simulink model "EPD629_WilliamsJ_AS08_Simulink"  (R2021b)
settings: Solver=VariableStepAuto  StartTime=0.0  StopTime=70  MaxStep=.02  RelTol=1e-3
values from neighbouring files (symbols this model uses):
  AirGasConstant_kJpkgK = 0.287    [EPD629_WilliamsJ_AS08.m]
  AirToFuelEquivalenceRatio_frac = 1    [EPD629_WilliamsJ_AS08.m]
  AmbientPressure_kPa = 98    [EPD629_WilliamsJ_AS08.m]
  BaseSparkAdvanceData_deg = min(MBTSparkAdvanceData_deg,BorderlineSparkAdvData_deg)    [EPD629_WilliamsJ_AS08.m]
  CrankAngleIVCToTDC_deg = 170    [EPD629_WilliamsJ_AS08.m]
  CylinderAirMassBreakpoints_mg = 0:25:400    [EPD629_WilliamsJ_AS08.m]
  DelayFuelInjectionToIVC_rev = 0.75    [EPD629_WilliamsJ_AS08.m]
  DelayFuelInjectionToIVCEst_rev = 0.75    [EPD629_WilliamsJ_AS08.m]
  DelayIVCToOxygenSensor_rev = 7    [EPD629_WilliamsJ_AS08.m]
  DischargeCoefficient_frac = 0.7    [EPD629_WilliamsJ_AS08.m]
  EngineDisplacement_L = 2.77    [EPD629_WilliamsJ_AS08.m]
  EngineInertia_kgm2 = 0.2    [EPD629_WilliamsJ_AS08.m]
  EngineMotoringFrictionData_Nm = Beta_0 + Beta_2*Omega_e.^2    [EPD629_WilliamsJ_AS08.m]
  EngineSpeedBreakpoints_rpm = 400:200:5000    [EPD629_WilliamsJ_AS08.m]
  FuelControlIntegralGain = 2e-5    (= 2e-05)    [EPD629_WilliamsJ_AS08.m]
  FuelControlProportionalGain = 5e-6    (= 5e-06)    [EPD629_WilliamsJ_AS08.m]
  FuelInjEvapTimeConstant_s = 0.8    [EPD629_WilliamsJ_AS08.m]
  FuelInjEvapTimeConstantEst_s = 0.8    [EPD629_WilliamsJ_AS08.m]
  FuelInjImpactFactor_frac = 0.3    [EPD629_WilliamsJ_AS08.m]
  FuelInjImpactFactorEst_frac = 0.3    [EPD629_WilliamsJ_AS08.m]
  FuelLowerHeatingValue_kJpkg = 44000    [EPD629_WilliamsJ_AS08.m]
  InletAirTemperature_K = 298    [EPD629_WilliamsJ_AS08.m]
  IntakeManifoldVolume_L = 5.8    [EPD629_WilliamsJ_AS08.m]
  ManifoldAirTemperature_K = 340    [EPD629_WilliamsJ_AS08.m]
  ManifoldPressureBreakpoints_kPa = 5:5:100    [EPD629_WilliamsJ_AS08.m]
  NumberOfCylinders = 6    [EPD629_WilliamsJ_AS08.m]
  OxygenSensorLambdaBP_frac = [0 0.9 0.92 0.94 0.96 0.985 0.999 1.001 1.015 1.04 1.06 1.08 1.1 2]    [EPD629_WilliamsJ_AS08.m]
  OxygenSensorSwitchSetpoint_mV = 450    [EPD629_WilliamsJ_AS08.m]
  OxygenSensorVoltageData_mV = [800 800 794 788 775 750 700 200 150 125 112 106 100 100]    [EPD629_WilliamsJ_AS08.m]
  SparkTorqFactorData_frac = 1 - (SparkTorqFactorRetFromMBTBP_deg.^2) /      (SparkTorqFactorRetFromMBTBP_deg(end)^2)    [EPD629_WilliamsJ_AS08.m]
  SparkTorqFactorRetFromMBTBP_deg = 0:5:45    [EPD629_WilliamsJ_AS08.m]
  StoichiometricAFR_frac = 14.7    [EPD629_WilliamsJ_AS08.m]
  ThermodynamicEfficiencyData_frac = Eta_0 + Eta_1*Omega_e + Eta_2*Omega_e.^2    [EPD629_WilliamsJ_AS08.m]
  ThrottleAreaBreakpoints_pct = ThrottleAreaData_pct    [EPD629_WilliamsJ_AS08.m]
  ThrottleAreaData_pct = 100 * ThrottleArea_mm2 / WideOpenThrottleArea_mm2    [EPD629_WilliamsJ_AS08.m]
  ThrottleFlowFunctionData_frac = PR.^(1/RatioOfSpecificHeats_frac) .*      sqrt( 2 * RatioOfSpecificHeats_frac / (RatioOfSpecificHeats_frac - 1) .*      (1 - PR.^((RatioOfSpecificHeats_frac - 1) / RatioOfSpecificHeats_frac)) )    [EPD629_WilliamsJ_AS08.m]
  ThrottleMassFlowCorrIntGain = 10    [EPD629_WilliamsJ_AS08.m]
  ThrottlePositionBreakpoints_pct = 0:100    [EPD629_WilliamsJ_AS08.m]
  ThrottlePositionData_pct = ThrottlePositionBreakpoints_pct    [EPD629_WilliamsJ_AS08.m]
  ThrottlePressureRatioBreakpoints_frac = 0:0.01:1    [EPD629_WilliamsJ_AS08.m]
  VECorrectionFactorIntGain = 0.02    [EPD629_WilliamsJ_AS08.m]
  WideOpenThrottleArea_mm2 = ThrottleArea_mm2(end)    [EPD629_WilliamsJ_AS08.m]
undefined symbols (not defined in the file or in its folder): MBTSparkAdvanceData_deg, SparkTorqFactorBreakpoints_frac, SparkTorqFactorRetFromMBTData_deg, VolumetricEfficiencyData_frac
(part 2 of 2)

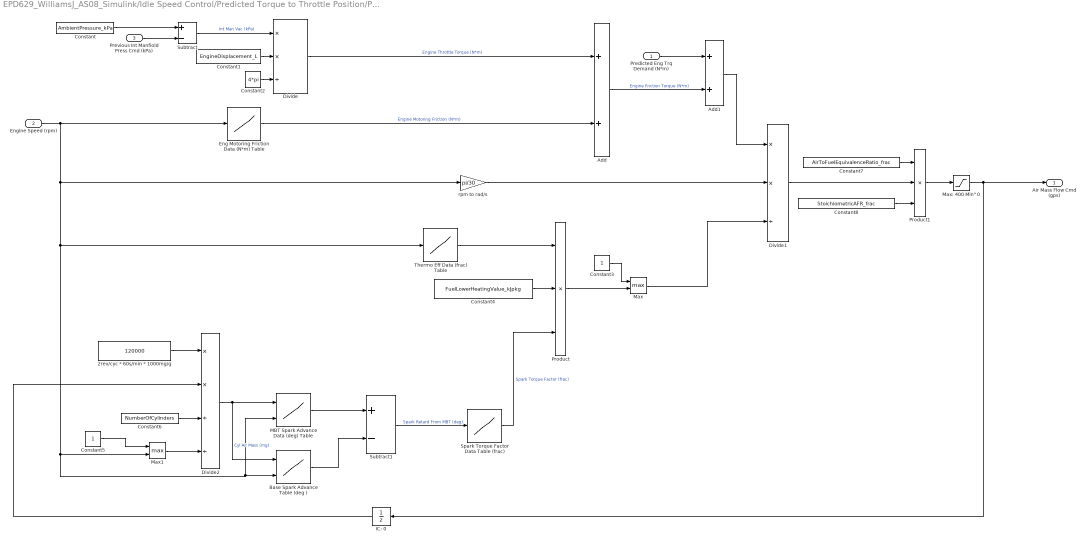
== system EPD629_WilliamsJ_AS08_Simulink/Idle Speed Control/Predicted Torque to Throttle Position/Predicted Torque to Air Mass Flow ==
  Predicted Eng Trq Demand (N*m) : Inport
  Engine Speed (rpm) : Inport  Port=2
  Previous Int Manfiold Press Cmd (kPa) : Inport  Port=3
  2rev/cyc * 60s/min * 1000mg/g : Constant  Value=120000
  Add : Sum
  Add1 : Sum
  Base Spark Advance Table (deg ) : Lookup_n-D  BreakpointsForDimension1=CylinderAirMassBreakpoints_mg  BreakpointsForDimension2=EngineSpeedBreakpoints_rpm  Table=BaseSparkAdvanceData_deg  ExtrapMethod=Clip  UseLastTableValue=on  InternalRulePriority=Speed  RndMeth=Simplest  InputSameDT=on
      settings: InputPortMap=u0,u1
  Constant : Constant  Value=AmbientPressure_kPa
  Constant1 : Constant  Value=EngineDisplacement_L
  Constant2 : Constant  Value=4*pi
  Constant3 : Constant
  Constant4 : Constant  Value=FuelLowerHeatingValue_kJpkg
  Constant5 : Constant
  Constant6 : Constant  Value=NumberOfCylinders
  Constant7 : Constant  Value=AirToFuelEquivalenceRatio_frac
  Constant8 : Constant  Value=StoichiometricAFR_frac
  Divide : Product  Inputs=**/
  Divide1 : Product  Inputs=**/
  Divide2 : Product  Inputs=**//
  Eng Motoring Friction Data (N*m) Table : Lookup_n-D  NumberOfTableDimensions=1  BreakpointsForDimension1=EngineSpeedBreakpoints_rpm  Table=EngineMotoringFrictionData_Nm  ExtrapMethod=Clip  UseLastTableValue=on  InternalRulePriority=Speed  RndMeth=Simplest  InputSameDT=on
  IC: 0 : UnitDelay  SampleTime=-1  HasFrameUpgradeWarning=on
  MBT Spark Advance Data (deg) Table : Lookup_n-D  BreakpointsForDimension1=CylinderAirMassBreakpoints_mg  BreakpointsForDimension2=EngineSpeedBreakpoints_rpm  Table=MBTSparkAdvanceData_deg  ExtrapMethod=Clip  UseLastTableValue=on  InternalRulePriority=Speed  RndMeth=Simplest  InputSameDT=on
      settings: InputPortMap=u0,u1
  Max : MinMax  Function=max  Inputs=2
  Max1 : MinMax  Function=max  Inputs=2
  "Max: 400 Min\" 0" : Saturate  UpperLimit=400  LowerLimit=0
  Product : Product  Inputs=3
  Product1 : Product  Inputs=3
  Spark Torque Factor Data Table (frac) : Lookup_n-D  NumberOfTableDimensions=1  BreakpointsForDimension1=SparkTorqFactorRetFromMBTBP_deg  Table=SparkTorqFactorData_frac  ExtrapMethod=Clip  UseLastTableValue=on  InternalRulePriority=Speed  RndMeth=Simplest  InputSameDT=on
  Subtract : Sum  Inputs=+-
  Subtract1 : Sum  Inputs=+-
  Thermo Eff Data (frac) Table : Lookup_n-D  NumberOfTableDimensions=1  BreakpointsForDimension1=EngineSpeedBreakpoints_rpm  Table=ThermodynamicEfficiencyData_frac  ExtrapMethod=Clip  UseLastTableValue=on  InternalRulePriority=Speed  RndMeth=Simplest  InputSameDT=on
  rpm to rad/s : Gain  Gain=pi/30
  Air Mass Flow Cmd (gps) : Outport
  wires:
  Previous Int Manfiold Press Cmd (kPa)/1 -> Subtract/2
  Constant/1 -> Subtract/1
  Subtract/1 -> Divide/1  "Int Man Vac (kPa)"
  Constant1/1 -> Divide/2
  Constant2/1 -> Divide/3
  Divide/1 -> Add/1  "Engine Throttle Torque (N*m)"
  Engine Speed (rpm)/1 -> rpm to rad/s/1, Thermo Eff Data (frac) Table/1, Max1/2, MBT Spark Advance Data (deg) Table/2, Base Spark Advance Table (deg )/2, Eng Motoring Friction Data (N*m) Table/1
  Eng Motoring Friction Data (N*m) Table/1 -> Add/2  "Engine Motoring Friction (N*m)"
  rpm to rad/s/1 -> Divide1/2
  Thermo Eff Data (frac) Table/1 -> Product/1
  Product/1 -> Max/2
  Constant3/1 -> Max/1
  Max/1 -> Divide1/3
  Constant4/1 -> Product/2
  Constant5/1 -> Max1/1
  Max1/1 -> Divide2/4
  Constant6/1 -> Divide2/3
  2rev/cyc * 60s/min * 1000mg/g/1 -> Divide2/1
  Divide1/1 -> Product1/2
  Constant7/1 -> Product1/1
  Constant8/1 -> Product1/3
  Product1/1 -> "Max: 400 Min\" 0"/1
  "Max: 400 Min\" 0"/1 -> IC: 0/1, Air Mass Flow Cmd (gps)/1
  IC: 0/1 -> Divide2/2
  Divide2/1 -> MBT Spark Advance Data (deg) Table/1, Base Spark Advance Table (deg )/1  "Cyl Air Mass (mg)"
  MBT Spark Advance Data (deg) Table/1 -> Subtract1/1
  Base Spark Advance Table (deg )/1 -> Subtract1/2
  Subtract1/1 -> Spark Torque Factor Data Table (frac)/1  "Spark Retard From MBT (deg)"
  Spark Torque Factor Data Table (frac)/1 -> Product/3  "Spark Torque Factor (frac)"
  Predicted Eng Trq Demand (N*m)/1 -> Add1/1
  Add/1 -> Add1/2  "Engine Friction Torque (N*m)"
  Add1/1 -> Divide1/1

== system EPD629_WilliamsJ_AS08_Simulink/SparkAndFuelControl/Spark Advance Control/Spark Advance Calculation ==
  Spark Retard from MBT (deg) : Inport
  Engine Speed (rpm) : Inport  Port=2
  SpeedDensityMassFlowEst_gps : Inport  Port=3
  Base Spark Advance Data (deg) Table : Lookup_n-D  BreakpointsForDimension1=CylinderAirMassBreakpoints_mg  BreakpointsForDimension2=EngineSpeedBreakpoints_rpm  Table=BaseSparkAdvanceData_deg  ExtrapMethod=Clip  UseLastTableValue=on  InternalRulePriority=Speed  RndMeth=Simplest  InputSameDT=on
      settings: InputPortMap=u0,u1
  Constant : Constant  Value=120000
  Constant1 : Constant  Value=NumberOfCylinders
  Constant2 : Constant
  Divide : Product  Inputs=**//
  MBT Spark Advance Data (deg) Table : Lookup_n-D  BreakpointsForDimension1=CylinderAirMassBreakpoints_mg  BreakpointsForDimension2=EngineSpeedBreakpoints_rpm  Table=MBTSparkAdvanceData_deg  ExtrapMethod=Clip  UseLastTableValue=on  InternalRulePriority=Speed  RndMeth=Simplest  InputSameDT=on
      settings: InputPortMap=u0,u1
  Max : MinMax  Function=max  Inputs=2
  Min : MinMax  Inputs=2
  Subtract : Sum  Inputs=+-
  Spark Advance (deg) : Outport
  wires:
  Engine Speed (rpm)/1 -> MBT Spark Advance Data (deg) Table/2, Base Spark Advance Data (deg) Table/2, Max/2
  Constant1/1 -> Divide/3
  Constant2/1 -> Max/1
  SpeedDensityMassFlowEst_gps/1 -> Divide/2
  Constant/1 -> Divide/1  "2rev/cyc * 60sec/min * 1000 mg/g"
  Max/1 -> Divide/4
  Base Spark Advance Data (deg) Table/1 -> Min/1  "Base Spark Advance (deg)"
  Divide/1 -> MBT Spark Advance Data (deg) Table/1, Base Spark Advance Data (deg) Table/1  "Cyl Air Mass (mg)"
  MBT Spark Advance Data (deg) Table/1 -> Subtract/1
  Spark Retard from MBT (deg)/1 -> Subtract/2
  Subtract/1 -> Min/2  "Spark Advance Max (deg)"
  Min/1 -> Spark Advance (deg)/1

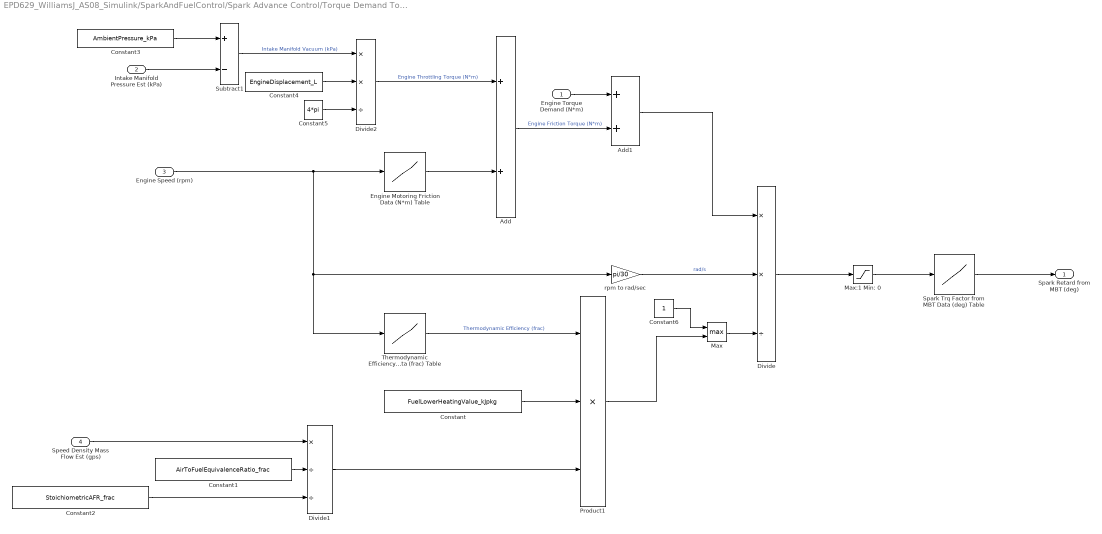
== system EPD629_WilliamsJ_AS08_Simulink/SparkAndFuelControl/Spark Advance Control/Torque Demand To Spark Retard from MBT ==
  Engine Torque Demand (N*m) : Inport
  Intake Manifold Pressure Est (kPa) : Inport  Port=2
  Engine Speed (rpm) : Inport  Port=3
  Speed Density Mass Flow Est (gps) : Inport  Port=4
  Add : Sum
  Add1 : Sum
  Constant : Constant  Value=FuelLowerHeatingValue_kJpkg
  Constant1 : Constant  Value=AirToFuelEquivalenceRatio_frac
  Constant2 : Constant  Value=StoichiometricAFR_frac
  Constant3 : Constant  Value=AmbientPressure_kPa
  Constant4 : Constant  Value=EngineDisplacement_L
  Constant5 : Constant  Value=4*pi
  Constant6 : Constant
  Divide : Product  Inputs=**/
  Divide1 : Product  Inputs=*//
  Divide2 : Product  Inputs=**/
  Engine Motoring Friction Data (N*m) Table : Lookup_n-D  NumberOfTableDimensions=1  BreakpointsForDimension1=EngineSpeedBreakpoints_rpm  Table=EngineMotoringFrictionData_Nm  ExtrapMethod=Clip  UseLastTableValue=on  InternalRulePriority=Speed  RndMeth=Simplest  InputSameDT=on
  Max : MinMax  Function=max  Inputs=2
  Max:1 Min: 0 : Saturate  UpperLimit=1  LowerLimit=0
  Product1 : Product  Inputs=3
  Spark Trq Factor from MBT Data (deg) Table : Lookup_n-D  NumberOfTableDimensions=1  BreakpointsForDimension1=SparkTorqFactorBreakpoints_frac  Table=SparkTorqFactorRetFromMBTData_deg  ExtrapMethod=Clip  UseLastTableValue=on  InternalRulePriority=Speed  RndMeth=Simplest  InputSameDT=on
  Subtract1 : Sum  Inputs=+-
  Thermodynamic Efficiency Data (frac) Table : Lookup_n-D  NumberOfTableDimensions=1  BreakpointsForDimension1=EngineSpeedBreakpoints_rpm  Table=ThermodynamicEfficiencyData_frac  ExtrapMethod=Clip  UseLastTableValue=on  InternalRulePriority=Speed  RndMeth=Simplest  InputSameDT=on
  rpm to rad/sec : Gain  Gain=pi/30
  Spark Retard from MBT (deg) : Outport
  wires:
  Engine Speed (rpm)/1 -> Engine Motoring Friction Data (N*m) Table/1, rpm to rad/sec/1, Thermodynamic Efficiency Data (frac) Table/1
  Divide2/1 -> Add/1  "Engine Throttling Torque (N*m)"
  Constant4/1 -> Divide2/2
  Constant3/1 -> Subtract1/1
  Intake Manifold Pressure Est (kPa)/1 -> Subtract1/2
  Subtract1/1 -> Divide2/1  "Intake Manifold Vacuum (kPa)"
  Constant5/1 -> Divide2/3
  Engine Motoring Friction Data (N*m) Table/1 -> Add/2
  Add/1 -> Add1/2  "Engine Friction Torque (N*m)"
  Engine Torque Demand (N*m)/1 -> Add1/1
  rpm to rad/sec/1 -> Divide/2  "rad/s"
  Add1/1 -> Divide/1
  Constant/1 -> Product1/2
  Thermodynamic Efficiency Data (frac) Table/1 -> Product1/1  "Thermodynamic Efficiency (frac)"
  Speed Density Mass Flow Est (gps)/1 -> Divide1/1
  Constant1/1 -> Divide1/2
  Constant2/1 -> Divide1/3
  Divide1/1 -> Product1/3
  Max/1 -> Divide/3
  Constant6/1 -> Max/1
  Product1/1 -> Max/2
  Divide/1 -> Max:1 Min: 0/1
  Max:1 Min: 0/1 -> Spark Trq Factor from MBT Data (deg) Table/1
  Spark Trq Factor from MBT Data (deg) Table/1 -> Spark Retard from MBT (deg)/1
